simulink model "bepf_balancing_scene"  (R2016b)
settings: Solver=VariableStepAuto  StartTime=0.0  StopTime=12  RelTol=1e-3
libraries: vrlib x3
settings Model: Creator=gagato  LastModifiedBy=gagato

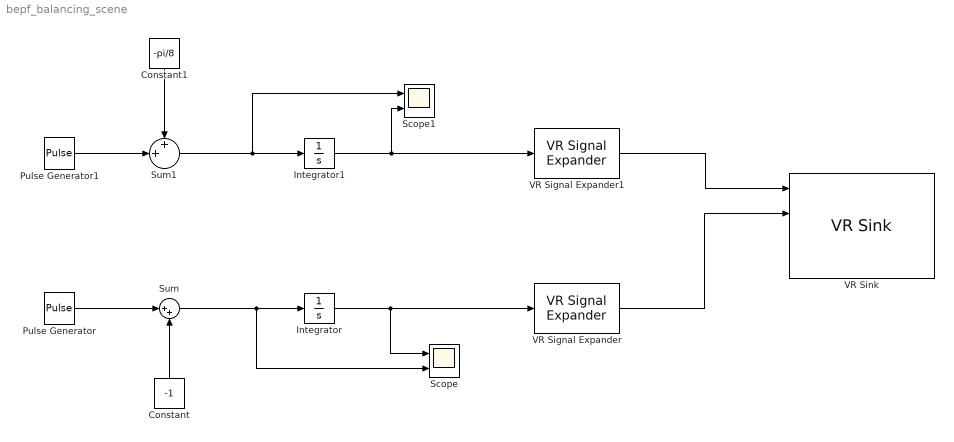
== system bepf_balancing_scene ==
  Constant : Constant  Value=-1
  Constant1 : Constant  Value=-pi/8
  Integrator : Integrator
  Integrator1 : Integrator
  Pulse Generator : DiscretePulseGenerator  PulseType=Time based  Amplitude=2  Period=6  PulseWidth=50  PhaseDelay=1.5
  Pulse Generator1 : DiscretePulseGenerator  PulseType=Time based  Amplitude=pi/4  Period=6  PulseWidth=50  PhaseDelay=1.5
  Scope : Scope  NumInputPorts=2
  Scope1 : Scope  NumInputPorts=2
  Sum : Sum  Inputs=|++
  Sum1 : Sum  Inputs=++|
  VR Signal Expander : vrlib/VR Signal Expander  outwidth=3  outidx=[1]
  VR Signal Expander1 : vrlib/VR Signal Expander  outwidth=4  outidx=[4]
  VR Sink : vrlib/VR Sink  InstantiateOnLoad=on  SampleTime=0.1  ViewEnable=on  RemoteChange=off  RemoteView=off  FieldsWritten=Bepf.rotation.4.1.1.double#Bepf.translation.3.1.1.double#bepf_kolo:1-37.rotation.4.1.1.double#bepf_kolo:2-38.rotation.4.1.1.double  WorldFileName=C:\Users\gagato\Documents\bepf\Matlab\bepf_balancing_scene.wrl  AutoView=on  VideoDimensions=[]  AllowVariableSize=off  FigureProperties="{'Position', 'Name', 'Viewpoint', 'CameraBound', 'CameraDirection', 'CameraPosition', 'CameraUpVector', 'ZoomFactor', 'Antialiasing', 'Headlight', 'Lighting', 'NavPanel', 'Sound', 'StatusBar', 'Stereo3D', 'Stereo3DCameraOffset', 'Stereo3DHIT', 'ToolBar', 'Textures', 'Transparency', 'Triad', 'Wireframe', 'NavZones', 'NavMode', 'NavSpeed', 'CaptureFileFormat', 'CaptureFileName', 'Record2DCompressMethod', 'Record2DCompressQuality', 'Record2D', 'Record2DFileName', 'Record2DFPS'; [9.3300000000000000e+02   1.2400000000000000e+02   5.7600000000000000e+02   3.5000000000000000e+02], '', 'General', 'on', [0.0000000000000000e+00   0.0000000000000000e+00  -1.0000000000000000e+00], [0.0000000000000000e+00   0.0000000000000000e+00   0.0000000000000000e+00], [0.0000000000000000e+00   1.0000000000000000e+00   0.0000000000000000e+00], [1.0000000000000000e+00], 'on', 'on', 'on', 'halfbar', 'on', 'on', 'off', [1.0000000149011612e-01], [0.0000000000000000e+00], 'on', 'on', 'on', 'none', 'off', 'off', 'fly', 'normal', 'tif', '%f_anim_%n.tif', 'auto', [7.5000000000000000e+01], 'off', '%f_anim_%n.avi', 'auto'}"
  wires:
  Sum/1 -> Integrator/1, Scope/2
  Constant/1 -> Sum/2
  Pulse Generator/1 -> Sum/1
  Integrator/1 -> VR Signal Expander/1, Scope/1
  Sum1/1 -> Scope1/1, Integrator1/1
  Integrator1/1 -> Scope1/2, VR Signal Expander1/1
  VR Signal Expander1/1 -> VR Sink/1
  VR Signal Expander/1 -> VR Sink/2
  Pulse Generator1/1 -> Sum1/2
  Constant1/1 -> Sum1/1
